simulink model "Visualization"  (R2026a)
settings: Solver=VariableStepAuto
undefined symbols (not defined in the file): ts_uav, waypoints
libraries: uavutilslib x1
settings Model: DataDictionary=QuadData.sldd  ModifiedByFormat=The MathWorks, Inc.  Creator=The MathWorks, Inc.  LastModifiedBy=The MathWorks, Inc.

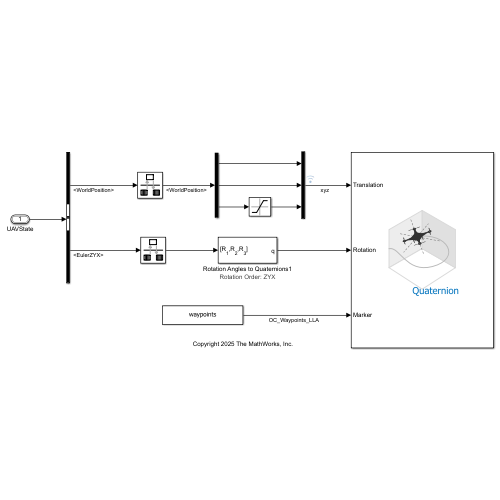
[thumbnail: Simulink's stored preview of the top-level diagram]
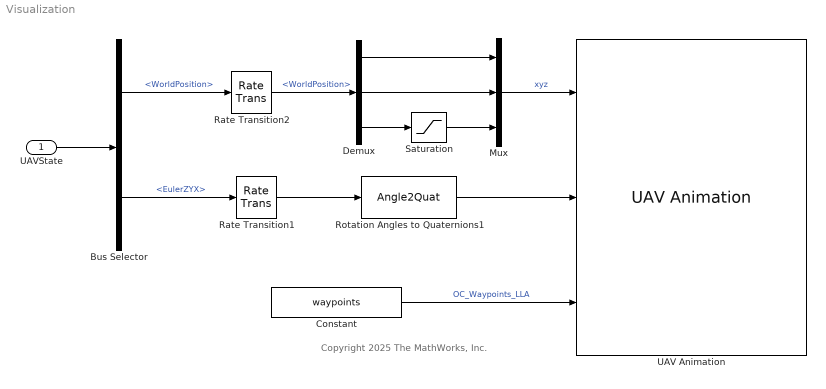
== system Visualization ==
  note: Copyright 2025 The MathWorks, Inc.
  UAVState : Inport  OutDataTypeStr=Bus: MultirotorGuidanceStateBus  SampleTime=0
  Bus Selector : BusSelector  OutputSignals=WorldPosition,EulerZYX
  Constant : Constant  Value=waypoints  SampleTime=ts_uav
  Demux : Demux  Outputs=3
  Mux : Mux  Inputs=3
  Rate Transition1 : RateTransition  Integrity=off  OutPortSampleTime=ts_uav
  Rate Transition2 : RateTransition  Integrity=off  OutPortSampleTime=ts_uav
  Rotation Angles to Quaternions1 : Angle2Quat
      settings: AttributesFormatString=Rotation Order: %<rotationOrder>
  Saturation : Saturate  UpperLimit=0.0001  LowerLimit=-inf
  UAV Animation : uavutilslib/UAV Animation  NumUAV=1  DynamicUAVConfig=off  UAVType=Multirotor  UAVSize=1  UAVColor=[1 0 0]  UAVTrajectoryAlpha=1  AlwaysShowAnimation=on  AxisLimits=[-Inf Inf;-Inf Inf;-Inf Inf]  TrajectoryBufferSize=100000  InertialZDirection=Down  RotationFormat=Quaternion  DrawMarkers=on  SampleTime=-1
  wires:
  Rate Transition1/1 -> Rotation Angles to Quaternions1/1
  Rotation Angles to Quaternions1/1 -> UAV Animation/2
  UAVState/1 -> Bus Selector/1
  Bus Selector/1 -> Rate Transition2/1  "<WorldPosition>"
  Bus Selector/2 -> Rate Transition1/1  "<EulerZYX>"
  Rate Transition2/1 -> Demux/1  "<WorldPosition>"
  Saturation/1 -> Mux/3
  Demux/2 -> Mux/2
  Demux/1 -> Mux/1
  Mux/1 -> UAV Animation/1  "xyz"
  Demux/3 -> Saturation/1
  Constant/1 -> UAV Animation/3  "OC_Waypoints_LLA"
